simulink model "Gear_Chain"  (R2013a)
settings: Solver=ode45  StartTime=0.0  StopTime=10.0  RelTol=1e-3
model workspace: external: MAT-File Gear_Chain.mat (data not in the file)
values from neighbouring files (symbols this model uses):
  ceffx = [0 78.53981625 157.0796325 230.383461 314.159265 366.5191425]    [Gear_Chain.mat]
  ceffy = [0.99 0.99 0.98 0.965 0.94 0.91]    [Gear_Chain.mat]
  Jc = 0    [Gear_Chain.mat]
  Jg = 0    [Gear_Chain.mat]
  Jm = 4.72    [Gear_Chain.mat]
  Jt = 1    [Gear_Chain.mat]
  Rg = evalin(sub,'Rg')    [Geal_val.m]    (also in Gear_Chain.mat = 2.09523809524)
settings Model: Creator=Nathan  LastModifiedBy=Nathan

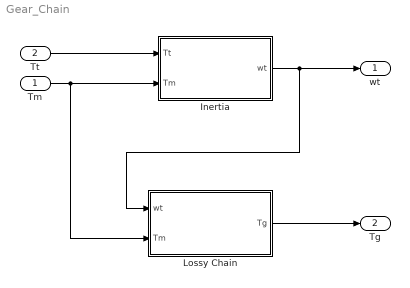
== system Gear_Chain ==
  Tm : Inport
  Tt : Inport  Port=2
  Inertia : Subsystem
  Lossy Chain : Subsystem
  wt : Outport
  Tg : Outport  Port=2
  wires:
  Tm/1 -> Lossy Chain/2(Tm), Inertia/2(Tm)
  Tt/1 -> Inertia/1(Tt)
  Inertia/1(wt) -> Lossy Chain/1(wt), wt/1
  Lossy Chain/1(Tg) -> Tg/1

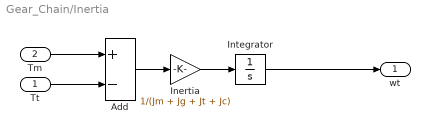
== system Gear_Chain/Inertia ==
  Tt : Inport
  Tm : Inport  Port=2
  Add : Sum  Inputs=+-
  Inertia : Gain  Gain=1/(Jm + Jg + Jt + Jc)
  Integrator : Integrator
  wt : Outport
  wires:
  Tt/1 -> Add/2
  Tm/1 -> Add/1
  Inertia/1 -> Integrator/1
  Integrator/1 -> wt/1
  Add/1 -> Inertia/1

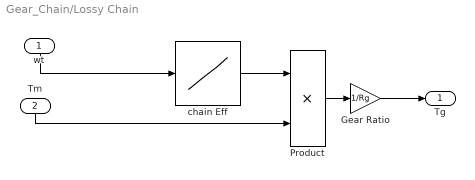
== system Gear_Chain/Lossy Chain ==
  wt : Inport
  Tm : Inport  Port=2
  Gear Ratio : Gain  Gain=1/Rg
  Product : Product
  chain Eff : Lookup_n-D  NumberOfTableDimensions=1  BreakpointsForDimension1=ceffx  Table=ceffy  RndMeth=Simplest  InputSameDT=on
  Tg : Outport
  wires:
  Tm/1 -> Product/2
  wt/1 -> chain Eff/1
  Product/1 -> Gear Ratio/1
  chain Eff/1 -> Product/1
  Gear Ratio/1 -> Tg/1
